simulink library "RgainzBtc"  (R2022b)
settings: Solver=VariableStepAuto  StartTime=0.0  StopTime=10.0  RelTol=1e-3
libraries: HandyTextFile x2, AudioStats x1
settings Model: Creator=kl13806  LastModifiedBy=kl13806
settings SolverCC: AlgebraicLoopSolver=TrustRegion
settings DebuggingCC: UnconnectedInputMsg=warning  UnconnectedOutputMsg=warning  UnconnectedLineMsg=warning  SFMachineParentedDataDiag=warning
settings ModelReferenceCC: EnableRefExpFcnMdlSchedulingChecks=on
settings RTWCC: DLArmComputeVersion=19.05

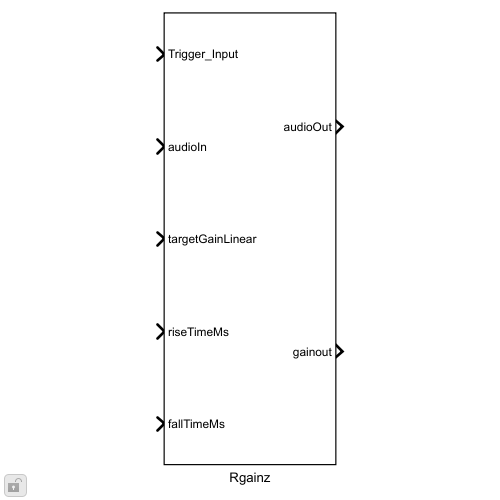
[thumbnail: Simulink's stored preview of the top-level diagram]
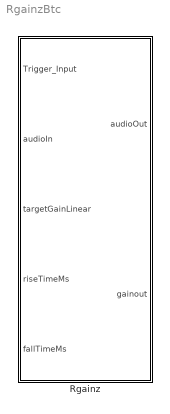
== system RgainzBtc ==
  Rgainz : Subsystem  mask(Chimes Rgainz){Config=[]}
      mask prompts: Config "RgainzConfig"
      mask init:
      | blkh=gcbh;
      | Config=BTConfig.Assert(blkh,Config);
      | [MASK_RAMPER_INIT, MASK_CURRENT_VAL_INIT]  = rgainzMask.Init ...
      |     (gcbh,Config.NumRampers,Config.InitialLinearGains);
      | Config.Validate();
      | 
      | %Flatten for MFB
      | MaskNumRampers = Config.NumRampers;

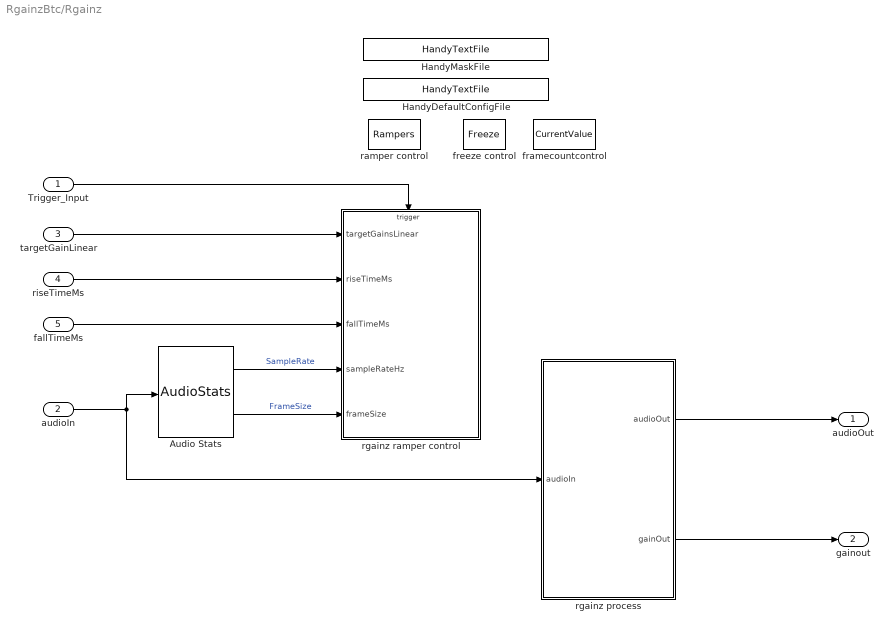
== system RgainzBtc/Rgainz ==
  Trigger_Input : Inport
  audioIn : Inport  Port=2
  targetGainLinear : Inport  Port=3
  riseTimeMs : Inport  Port=4
  fallTimeMs : Inport  Port=5
  Audio Stats : AudioStats/AudioStats  DoSampleRate=on  TypeSampleRate=single  DoCallRate=off  TypeCallRate=Inherit: auto  DoFrameSize=on  TypeFrameSize=single  DoChannelCount=off  TypeChannelCount=Inherit: auto  DoTaskRateFactor=off  TypeTaskRateFactor=Inherit: auto  MacroNameRoot=AUDIO  MacroNameRootEval='AUDIO'  IsMacroNameEval=off  MacroSampleRate=off  MacroCallRate=off  MacroFrameSize=off  MacroChannelCount=off  MacroTaskRateFactor=off  MacroTaskId=off  ValidateSampleRate=off  ValueSampleRate=[]  ValidateCallRate=off  ValueCallRate=[]  ValidateFrameSize=off  ValueFrameSize=[]  ValidateChannelCount=off  ValueChannelCount=[]  ValidateTaskRateFactor=off  ValueTaskRateFactor=[]
  HandyDefaultConfigFile : HandyTextFile/HandyTextFile  TemplateSource=Config  FileSuffix=Init  OpenDialogOnLoad=off  UseThisBlockName=off  TheDefaultText=|  ShowInLibBrowser=on
      | % $(FILENAME) Setup model parameters for each "Init" callback (e.g. update diagram)
      | sample_rate_in_hertz = 44100;
      | frame_size = 32;
      | sysin_channel_count = 2;
  HandyMaskFile : HandyTextFile/HandyTextFile  TemplateSource=Mask  FileSuffix=Init  OpenDialogOnLoad=off  UseThisBlockName=off  TheDefaultText=|  ShowInLibBrowser=on
      | % $(FILENAME) Setup model parameters for each "Init" callback (e.g. update diagram)
      | sample_rate_in_hertz = 44100;
      | frame_size = 32;
      | sysin_channel_count = 2;
  framecountcontrol : DataStoreMemory  DataStoreName=CurrentValue  InitialValue=zeros(1,Config.NumRampers)  ShowAdditionalParam=off  OutDataTypeStr=Bus: rgainz_bus
  freeze control : DataStoreMemory  DataStoreName=Freeze  InitialValue=zeros(1,Config.NumRampers)  ShowAdditionalParam=off  OutDataTypeStr=uint32
  ramper control : DataStoreMemory  DataStoreName=Rampers  InitialValue=zeros(1,Config.NumRampers)  ShowAdditionalParam=off  OutDataTypeStr=Bus: rgainz_bus
  rgainz process : MATLAB Function  TreatAsAtomicUnit=on
  rgainz ramper control : MATLAB Function  TreatAsAtomicUnit=on
  audioOut : Outport  VectorParamsAs1DForOutWhenUnconnected=off
  gainout : Outport  Port=2  VectorParamsAs1DForOutWhenUnconnected=off
  wires:
  audioIn/1 -> rgainz process/1(audioIn), Audio Stats/1
  targetGainLinear/1 -> rgainz ramper control/1(targetGainsLinear)
  riseTimeMs/1 -> rgainz ramper control/2(riseTimeMs)
  fallTimeMs/1 -> rgainz ramper control/3(fallTimeMs)
  Audio Stats/1 -> rgainz ramper control/4(sampleRateHz)  "SampleRate"
  Audio Stats/2 -> rgainz ramper control/5(frameSize)  "FrameSize"
  Trigger_Input/1 -> rgainz ramper control/Trigger
  rgainz process/1(audioOut) -> audioOut/1
  rgainz process/2(gainOut) -> gainout/1

== matlab function RgainzBtc/Rgainz/rgainz process ==
  data: audioIn input; audioOut output; MaskNumRampers parameter; Freeze data_store_memory; Rampers data_store_memory; CurrentValue data_store_memory; gainOut output
function [audioOut, gainOut] = rgainz_process(audioIn, MaskNumRampers) 
    %#codegen
    % Description: Check whether the block is in the Rise or Fall phase and
    % apply the corresponding ramp coefficient.
    
    global Rampers;
    global CurrentValue;

    % Set the size of the output buffer
    audioOut = coder.nullcopy(audioIn);
    gainOut=single(zeros(1,MaskNumRampers));
    gain=single(zeros(1,MaskNumRampers));
    [frame_size,~] = size(audioIn);

    % Loop through rampers and apply their gain coefficients
    k = single( ones( 1, MaskNumRampers ));
    for ramper = 1:MaskNumRampers
        % Check whether in Rise or Fall phase in order to apply the
        % corresponding ramp coefficient
        [CurrentValue(ramper).isRisePhase,CurrentValue(ramper).isFallPhase] = check_phase(CurrentValue(ramper));
        k(ramper) = single( 1.0 );

        % Ensure the lowest gain is at -100 dB or 1e-5 linear
        gain(ramper) = max(CurrentValue(ramper).currentGain, 1e-5);
        if ( CurrentValue(ramper).isRisePhase == 1 ) && ( CurrentValue(ramper).riseFrameCount > 0 )
            k(ramper) = Rampers(ramper).riseRampCoeff;
            CurrentValue(ramper).riseFrameCount = CurrentValue(ramper).riseFrameCount - 1;
        elseif ( CurrentValue(ramper).isFallPhase == 1 ) && ( CurrentValue(ramper).fallFrameCount > 0 )
            k(ramper) = Rampers(ramper).fallRampCoeff;
            CurrentValue(ramper).fallFrameCount = CurrentValue(ramper).fallFrameCount - 1;
        end

        % Update the current gain so that the ramping occurs smoothly 
        % across consecutive frames
        % Loop through samples apply gain to channels
        for n=1:frame_size
             gain(ramper) = gain(ramper) * k(ramper);
             audioOut(n,ramper) = audioIn(n,ramper)* gain(ramper);
        end

        % Check if ramp up finishes early
        if(( CurrentValue(ramper).isRisePhase == 1          ) && ...
           ( gain(ramper) > CurrentValue(ramper).targetGain ) && ...
           ( CurrentValue(ramper).riseFrameCount ~= 0       ))        
           CurrentValue(ramper).riseFrameCount = int32(0);
        end 

        % Check if ramp down finishes early
        if(( CurrentValue(ramper).isFallPhase == 1          ) && ...
           ( gain(ramper) < CurrentValue(ramper).targetGain ) && ...
           ( CurrentValue(ramper).fallFrameCount ~= 0       ))        
            CurrentValue(ramper).fallFrameCount = int32(0);
        end    

        % Check if ramping done
        riseDone = ( CurrentValue(ramper).isRisePhase == 1 ) && ( CurrentValue(ramper).riseFrameCount == 0 );
        fallDone = ( CurrentValue(ramper).isFallPhase == 1 ) && ( CurrentValue(ramper).fallFrameCount == 0 );
        [gain(ramper),CurrentValue(ramper)] = check_ramp_done(riseDone, fallDone, gain(ramper),CurrentValue(ramper));                     
        
        % Update current gain for the next frame
        CurrentValue(ramper).currentGain = gain(ramper);
        gainOut(ramper) = CurrentValue(ramper).currentGain;
    end
end

function [isRisePhase, isFallPhase] = check_phase(CurrentValue)
    % Check which phase is in progress based on the current and target
    % gains. If they are both equal, then there is no need for any change.
    if ((( CurrentValue.currentGain < CurrentValue.targetGain )) && ( CurrentValue.riseFrameCount > 0 ))        
        isRisePhase = int32(1);
        isFallPhase = int32(0);
    elseif ((( CurrentValue.targetGain < CurrentValue.currentGain )) && ( CurrentValue.fallFrameCount > 0 ))
        isRisePhase = int32(0);
        isFallPhase = int32(1);
    else
        isRisePhase = int32(0);
        isFallPhase = int32(0);
    end
end

function [gain,CurrentValue] = check_ramp_done(riseDone, fallDone, gain, CurrentValue)
    % Check if ramping is complete
    if riseDone || fallDone
        gain = CurrentValue.targetGain;
        CurrentValue.isRisePhase = int32(0);
        CurrentValue.isFallPhase = int32(0);
    end
end

== matlab function RgainzBtc/Rgainz/rgainz ramper control ==
  data targetGainsLinear settings: description=This vector signal must provide a linear target gain for every ramper.
  data riseTimeMs settings: description="If provided (i.e. non zero), this argument causes the \"ramp times (ms)\" input to be ignored. The block will calculate ramp times itself to ensure all gain changes happen at the db_per_sec slope provided."
  data fallTimeMs settings: description=|
      | The rampTimes_ms signal can accept one or more ramp times. If only one time is given, it is applied to all rampers. When more than one time is given, the times are delt out to the rampers in order. If not enough times are specified to cover all the rampers, the last given time is filled in to any remaining rampers.
      | NOTE: this input signal is entirely ignored if the db_per_sec input signal is non-zero. Attach the db_per_sec input to a ground block if you want to provide ramp times via this input.
  data sampleRateHz settings: description="This input is required for control calculations to work. The \"Audio Stats\" block is a handy tool to lift this property right off an inbound audio signal and feed it to this block automatically without using workspace parameters or other constants."
  data frameSize settings: description="This input is required for control calculations to work. The \"Audio Stats\" block is a handy tool to lift this property right off an inbound audio signal and feed it to this block automatically without using workspace parameters or other constants."
  data: targetGainsLinear input size=[1 MaskNumRampers]; riseTimeMs input; fallTimeMs input; sampleRateHz input; frameSize input; MaskNumRampers parameter; Freeze data_store_memory; Rampers data_store_memory; CurrentValue data_store_memory
  events: trigger input FUNCTION_CALL_EVENT
function control(...
     targetGainsLinear, riseTimeMs, fallTimeMs, ...
     sampleRateHz, frameSize, MaskNumRampers)

global Freeze;
global Rampers;
global CurrentValue;

rgain_SILENT_GAIN = RgainBusUtil.GetSilentGainLinear();

% Get the sizes of the provided target and time specifications
numGains = numel(targetGainsLinear);

% Step 1: FREEZE the gain ramper so that we can perform calculations based
% on the current gain value.

for ramper=1:MaskNumRampers
    Freeze(ramper) = uint32(1); % freeze the gain
    % assign gains and ramp times
    targetGain = single(targetGainsLinear(mod(ramper-1,numGains)+1));

    % Step 2: Nudge the gain values a bit if they are sitting at zero.
    % When this control set goes live, ensure that the current gain will move.
    % If current gain is zero, replace with a value very close to zero. What we
    % really want is a value which is on the edge of perception - not too small
    % or large. If the value is too small, we'll waste some of our ramp time
    % in perceived silence. If the value is too large, the audio will lurch
    % into perceptability at the start of the ramp.
    currentGain = max(CurrentValue(ramper).currentGain, rgain_SILENT_GAIN);
    targetGain  = max(targetGain, rgain_SILENT_GAIN);
    
    % Step 3b: QUANTIZE the desired ramp time to our FrameSize. Also retrieve 
    % the whole number of frames required to best match requested ramp time.
    % Ensure that at least one frame is used. The frame size will therefore
    % determine the steepest ramp (i.e. within one frame you can go anywhere).
    quantumMs = 1000 * frameSize / sampleRateHz;
    riseNumFrames = riseTimeMs(ramper) / quantumMs;
    riseNumFrames = max (1, ceil(riseNumFrames));
%    quantizedRiseTimeMs = riseNumFrames * quantumMs;

    fallNumFrames = fallTimeMs(ramper) / quantumMs;
    fallNumFrames = max (1, ceil(fallNumFrames));
%    quantizedFallTimeMs = fallNumFrames * quantumMs;
    
%     onNumFrames = onTimeMs / quantumMs;
%     onNumFrames = max (1, round(onNumFrames));
%     
%     offNumFrames = offTimeMs / quantumMs;
%     offNumFrames = max (1, round(offNumFrames));
    
    % In order to have the desired ramp time, the slope must vary dependent
    % on the gain differencebetween target and current value.
    % Ramper's coefficient is therefore calculated as follows:
    %
    %   TargetGain = CurrentGain *( RampCoef ^ (Fs*RampTime_ms/1000) )
    %
    % therefore...
    %
    %                     log(TargetGain/CurrentGain)
    %   log(RampCoef) = ------------------------------
    %                        Fs*(RampTime_ms/1000)
    %
    
    % RAVI
    isRisePhase = 0;
    isFallPhase = 0;
    if ( abs( targetGain - currentGain ) <= rgain_SILENT_GAIN )
      riseRampCoeff = single(1.0);
      fallRampCoeff = single(1.0);
    else
      factor = ( targetGain / currentGain );
      if ( factor >= 1.0 )
          isRisePhase = 1;
          isFallPhase = 0;
      else
          isRisePhase = 0;
          isFallPhase = 1;
      end
      if ( factor < 1.0 )
          factor = 1.0 / factor;
      end
      factor_log = log( factor );
%      riseRampCoeff = exp( factor_log / (sampleRateHz * quantizedRiseTimeMs / 1000));
%      fallRampCoeff = exp(-1*factor_log / (sampleRateHz * quantizedFallTimeMs / 1000));
      riseRampCoeff = exp( factor_log / ( riseNumFrames * frameSize ));
      fallRampCoeff = exp(-1*factor_log / ( fallNumFrames * frameSize ));
    end

    % Output control signals    
    Rampers(ramper).riseFrameCount = int32(riseNumFrames);
    Rampers(ramper).fallFrameCount = int32(fallNumFrames);
    Rampers(ramper).riseRampCoeff  = single(riseRampCoeff);
    Rampers(ramper).fallRampCoeff  = single(fallRampCoeff);
%   Rampers(ramper).onFrameCount   = int32(onNumFrames);
%   Rampers(ramper).offFrameCount  = int32(offNumFrames);    
    Rampers(ramper).targetGain     = single(targetGainsLinear(ramper));
    Rampers(ramper).currentGain    = single(currentGain);
    Rampers(ramper).isRisePhase    = int32( isRisePhase );
    Rampers(ramper).isFallPhase    = int32( isFallPhase );
    
    % Initializing the current value. This global variable will be updated
    % so that multiple cycles of ON-OFF can occur.
    CurrentValue(ramper) = Rampers(ramper);
    Freeze(ramper) = Freeze(ramper) - uint32(1);
end
